simulink model "TST_BrkPed_SetData"  (R2016b)
settings: Solver=FixedStepDiscrete  StartTime=0.0  StopTime=simTime  FixedStep=sampleTime  RelTol=1e-3
values from neighbouring files (symbols this model uses):
  testCase = 1    [initTST_BrkPed_SetData_001.m]
libraries: simulink x4, UnitTest_Lib x2
settings Model: Creator=zhengjinyan  LastModifiedBy=zhengjinyan
settings DebuggingCC: SignalRangeChecking=error

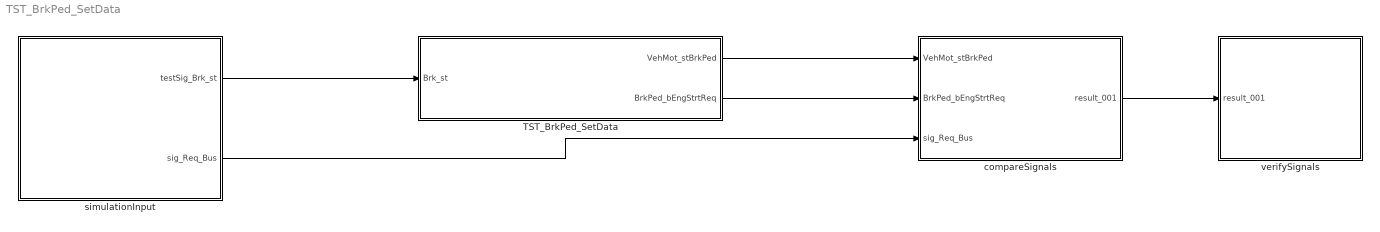
== system TST_BrkPed_SetData ==
  TST_BrkPed_SetData : Subsystem
  compareSignals : Subsystem
  simulationInput : Subsystem
  verifySignals : Subsystem
  wires:
  simulationInput/1(testSig_Brk_st) -> TST_BrkPed_SetData/1(Brk_st)
  TST_BrkPed_SetData/1(VehMot_stBrkPed) -> compareSignals/1(VehMot_stBrkPed)
  TST_BrkPed_SetData/2(BrkPed_bEngStrtReq) -> compareSignals/2(BrkPed_bEngStrtReq)
  simulationInput/2(sig_Req_Bus) -> compareSignals/3(sig_Req_Bus)
  compareSignals/1(result_001) -> verifySignals/1(result_001)

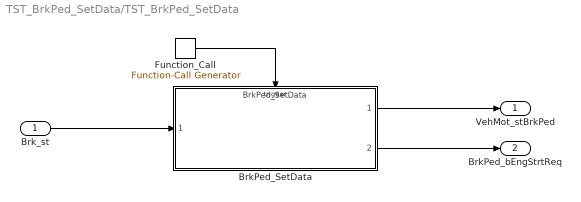
== system TST_BrkPed_SetData/TST_BrkPed_SetData ==
  Brk_st : Inport
  BrkPed_SetData : ModelReference  ModelNameDialog=BrkPed_SetData  SimulationMode=Normal  ModelReferenceVersion=1.4  TriggerPortName=function  TriggerPortTriggerType=function-call  TriggerPortStatesWhenEnabling=held
  Function_Call : simulink/Ports & Subsystems/Function-Call Generator  sample_time=sampleTime  numberOfIterations=1
  VehMot_stBrkPed : Outport
  BrkPed_bEngStrtReq : Outport  Port=2
  wires:
  Function_Call/1 -> BrkPed_SetData/Trigger
  Brk_st/1 -> BrkPed_SetData/1
  BrkPed_SetData/1 -> VehMot_stBrkPed/1
  BrkPed_SetData/2 -> BrkPed_bEngStrtReq/1

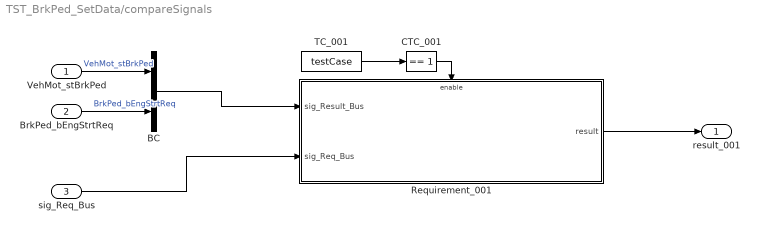
== system TST_BrkPed_SetData/compareSignals ==
  VehMot_stBrkPed : Inport
  BrkPed_bEngStrtReq : Inport  Port=2
  sig_Req_Bus : Inport  Port=3
  BC : BusCreator  Inputs=2
  CTC_001 : simulink/Logic and Bit Operations/Compare To Constant  relop===  const=1  OutDataTypeStr=boolean
  Requirement_001 : Subsystem
  TC_001 : Constant  Value=testCase
  result_001 : Outport
  wires:
  VehMot_stBrkPed/1 -> BC/1  "VehMot_stBrkPed"
  BrkPed_bEngStrtReq/1 -> BC/2  "BrkPed_bEngStrtReq"
  TC_001/1 -> CTC_001/1
  CTC_001/1 -> Requirement_001/Enable
  sig_Req_Bus/1 -> Requirement_001/2(sig_Req_Bus)
  BC/1 -> Requirement_001/1(sig_Result_Bus)
  Requirement_001/1(result) -> result_001/1

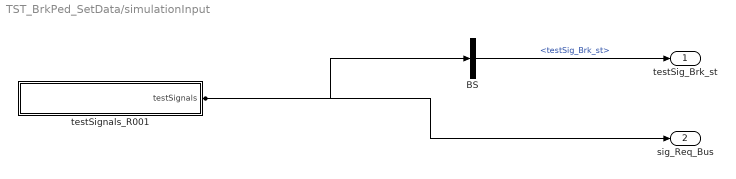
== system TST_BrkPed_SetData/simulationInput ==
  BS : BusSelector  OutputSignals=testSig_Brk_st
  testSignals_R001 : Subsystem
  testSig_Brk_st : Outport
  sig_Req_Bus : Outport  Port=2
  wires:
  BS/1 -> testSig_Brk_st/1  "<testSig_Brk_st>"
  testSignals_R001/1(testSignals) -> BS/1, sig_Req_Bus/1

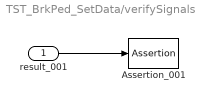
== system TST_BrkPed_SetData/verifySignals ==
  result_001 : Inport
  Assertion_001 : Assertion  Enabled=off
  wires:
  result_001/1 -> Assertion_001/1

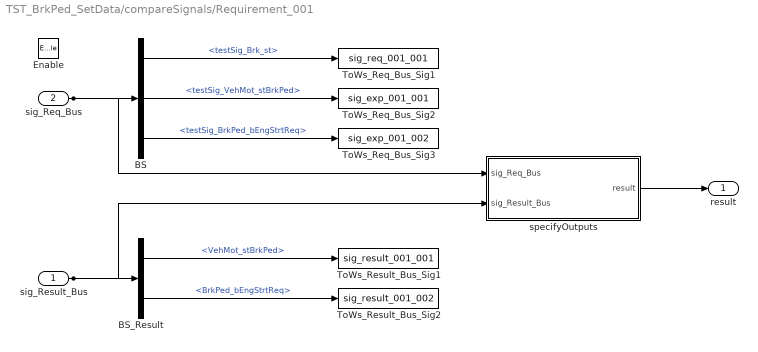
== system TST_BrkPed_SetData/compareSignals/Requirement_001 ==
  sig_Result_Bus : Inport
  sig_Req_Bus : Inport  Port=2
  Enable : EnablePort
  BS : BusSelector  OutputSignals=testSig_Brk_st,testSig_VehMot_stBrkPed,testSig_BrkPed_bEngStrtReq
  BS_Result : BusSelector  OutputSignals=VehMot_stBrkPed,BrkPed_bEngStrtReq
  ToWs_Req_Bus_Sig1 : ToWorkspace  VariableName=sig_req_001_001  SaveFormat=Structure With Time
  ToWs_Req_Bus_Sig2 : ToWorkspace  VariableName=sig_exp_001_001  SaveFormat=Structure With Time
  ToWs_Req_Bus_Sig3 : ToWorkspace  VariableName=sig_exp_001_002  SaveFormat=Structure With Time
  ToWs_Result_Bus_Sig1 : ToWorkspace  VariableName=sig_result_001_001  SaveFormat=Structure With Time
  ToWs_Result_Bus_Sig2 : ToWorkspace  VariableName=sig_result_001_002  SaveFormat=Structure With Time
  specifyOutputs : Subsystem
  result : Outport
  wires:
  sig_Req_Bus/1 -> BS/1, specifyOutputs/1(sig_Req_Bus)
  BS/1 -> ToWs_Req_Bus_Sig1/1  "<testSig_Brk_st>"
  BS/2 -> ToWs_Req_Bus_Sig2/1  "<testSig_VehMot_stBrkPed>"
  BS/3 -> ToWs_Req_Bus_Sig3/1  "<testSig_BrkPed_bEngStrtReq>"
  sig_Result_Bus/1 -> BS_Result/1, specifyOutputs/2(sig_Result_Bus)
  BS_Result/1 -> ToWs_Result_Bus_Sig1/1  "<VehMot_stBrkPed>"
  BS_Result/2 -> ToWs_Result_Bus_Sig2/1  "<BrkPed_bEngStrtReq>"
  specifyOutputs/1(result) -> result/1

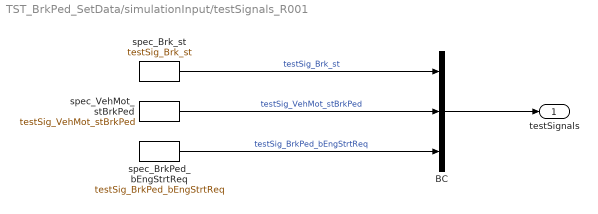
== system TST_BrkPed_SetData/simulationInput/testSignals_R001 ==
  BC : BusCreator  Inputs=3
  spec_BrkPed_bEngStrtReq : FromWorkspace  VariableName=testSig_BrkPed_bEngStrtReq  Interpolate=off  OutputAfterFinalValue=Holding final value
  spec_Brk_st : FromWorkspace  VariableName=testSig_Brk_st  Interpolate=off  OutputAfterFinalValue=Holding final value
  spec_VehMot_stBrkPed : FromWorkspace  VariableName=testSig_VehMot_stBrkPed  Interpolate=off  OutputAfterFinalValue=Holding final value
  testSignals : Outport
  wires:
  BC/1 -> testSignals/1
  spec_Brk_st/1 -> BC/1  "testSig_Brk_st"
  spec_VehMot_stBrkPed/1 -> BC/2  "testSig_VehMot_stBrkPed"
  spec_BrkPed_bEngStrtReq/1 -> BC/3  "testSig_BrkPed_bEngStrtReq"

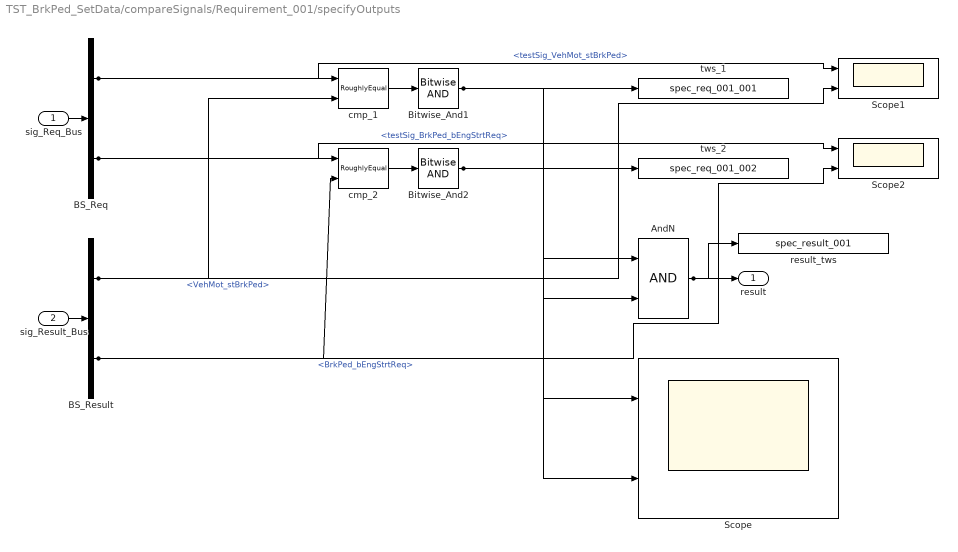
== system TST_BrkPed_SetData/compareSignals/Requirement_001/specifyOutputs ==
  sig_Req_Bus : Inport
  sig_Result_Bus : Inport  Port=2
  AndN : Logic
  BS_Req : BusSelector  OutputSignals=testSig_VehMot_stBrkPed,testSig_BrkPed_bEngStrtReq
  BS_Result : BusSelector  OutputSignals=VehMot_stBrkPed,BrkPed_bEngStrtReq
  Bitwise_And1 : simulink/Logic and Bit Operations/Bitwise Operator  logicop=AND  UseBitMask=off  BitMask=bin2dec('11011001')  BitMaskRealWorld=Stored Integer
  Bitwise_And2 : simulink/Logic and Bit Operations/Bitwise Operator  logicop=AND  UseBitMask=off  BitMask=bin2dec('11011001')  BitMaskRealWorld=Stored Integer
  Scope : Scope  NumInputPorts=2
  Scope1 : Scope  NumInputPorts=2
  Scope2 : Scope  NumInputPorts=2
  cmp_1 : UnitTest_Lib/RoughlyEqual  slope=0.1
  cmp_2 : UnitTest_Lib/RoughlyEqual  slope=0.1
  result_tws : ToWorkspace  VariableName=spec_result_001
  tws_1 : ToWorkspace  VariableName=spec_req_001_001
  tws_2 : ToWorkspace  VariableName=spec_req_001_002
  result : Outport
  wires:
  sig_Req_Bus/1 -> BS_Req/1
  sig_Result_Bus/1 -> BS_Result/1
  AndN/1 -> result/1, result_tws/1
  BS_Req/1 -> cmp_1/1, Scope1/1  "<testSig_VehMot_stBrkPed>"
  BS_Result/1 -> cmp_1/2, Scope1/2  "<VehMot_stBrkPed>"
  cmp_1/1 -> Bitwise_And1/1
  Bitwise_And1/1 -> tws_1/1, AndN/1, Scope/1
  BS_Req/2 -> cmp_2/1, Scope2/1  "<testSig_BrkPed_bEngStrtReq>"
  BS_Result/2 -> cmp_2/2, Scope2/2  "<BrkPed_bEngStrtReq>"
  cmp_2/1 -> Bitwise_And2/1
  Bitwise_And2/1 -> tws_2/1, AndN/2, Scope/2
